simulink model "Lecture_3_Exercises_Simulink"  (R2023b)
settings: Solver=VariableStepAuto  StartTime=0.0  StopTime=10.0  RelTol=1e-3
values from neighbouring files (symbols this model uses):
  Kd = 0.25    [Lecture_3_Exercises.m]
  Ki = 0.05    [Lecture_3_Exercises.m]
  Kp = 0.5    [Lecture_3_Exercises.m]
  P = theta/delta    [Lecture_3_Exercises.m]
settings Model: Creator=therk  LastModifiedBy=therk

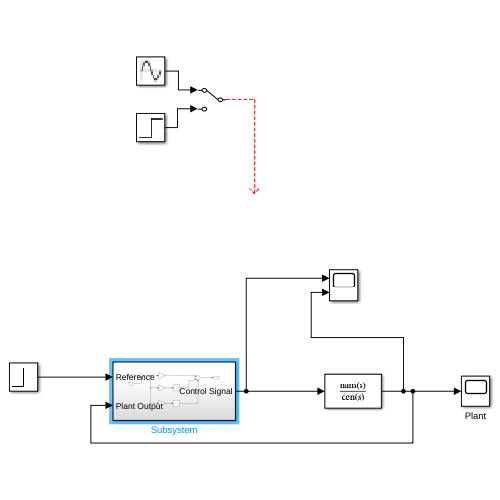
[thumbnail: Simulink's stored preview of the top-level diagram]
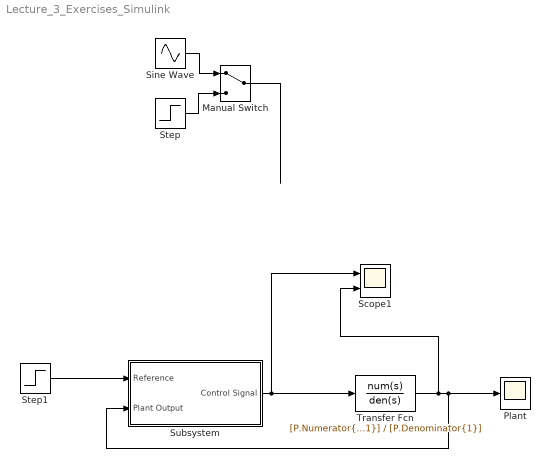
== system Lecture_3_Exercises_Simulink ==
  Manual Switch : ManualSwitch
  Plant : Scope
  Scope1 : Scope  NumInputPorts=2
  Sine Wave : Sin  Frequency=0.244  SampleTime=0
  Step : Step  SampleTime=0
  Step1 : Step  SampleTime=0
  Subsystem : Subsystem
  Transfer Fcn : TransferFcn  Numerator=[P.Numerator{1}]  Denominator=[P.Denominator{1}]
  wires:
  Sine Wave/1 -> Manual Switch/1
  Step/1 -> Manual Switch/2
  Step1/1 -> Subsystem/1(Reference)
  Transfer Fcn/1 -> Scope1/2, Subsystem/2(Plant Output), Plant/1
  Manual Switch/1 -> ?
  Subsystem/1(Control Signal) -> Transfer Fcn/1, Scope1/1

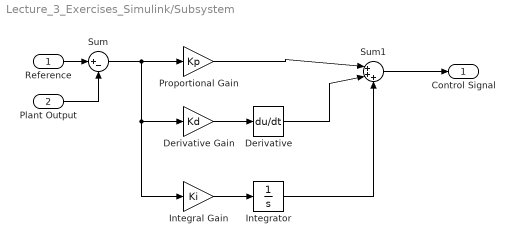
== system Lecture_3_Exercises_Simulink/Subsystem ==
  Reference : Inport
  Plant Output : Inport  Port=2
  Derivative : Derivative
  Derivative Gain : Gain  Gain=Kd
  Integral Gain : Gain  Gain=Ki
  Integrator : Integrator
  Proportional Gain : Gain  Gain=Kp
  Sum : Sum  Inputs=|+-
  Sum1 : Sum  Inputs=|+++
  Control Signal : Outport
  wires:
  Proportional Gain/1 -> Sum1/1
  Derivative Gain/1 -> Derivative/1
  Derivative/1 -> Sum1/2
  Sum1/1 -> Control Signal/1
  Integral Gain/1 -> Integrator/1
  Integrator/1 -> Sum1/3
  Plant Output/1 -> Sum/2
  Reference/1 -> Sum/1
  Sum/1 -> Integral Gain/1, Derivative Gain/1, Proportional Gain/1
